simulink model "untitled"  (R2014b)
settings: Solver=ode45  StartTime=0.0  StopTime=10.0  RelTol=1e-3
settings Model: Creator=maksimka  LastModifiedBy=maksimka

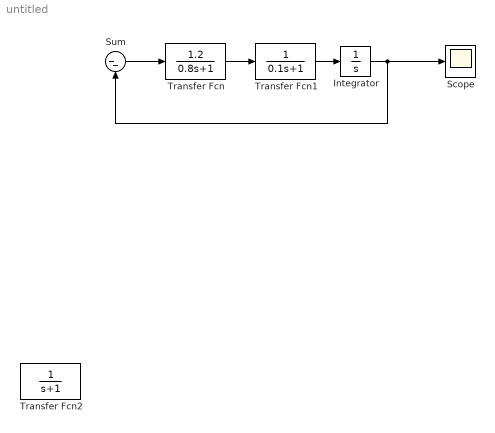
== system untitled ==
  Integrator : Integrator
  Scope : Scope
  Sum : Sum  Inputs=|--
  Transfer Fcn : TransferFcn  Numerator=[1.2]  Denominator=[0.8 1]
  Transfer Fcn1 : TransferFcn  Denominator=[0.1 1]
  Transfer Fcn2 : TransferFcn  Denominator=[1 1]
  wires:
  Transfer Fcn/1 -> Transfer Fcn1/1
  Transfer Fcn1/1 -> Integrator/1
  Integrator/1 -> Sum/2, Scope/1
  Sum/1 -> Transfer Fcn/1
